simulink model "MPCtest1"  (Simulink 10.0)
settings: Solver=VariableStepDiscrete  StartTime=0.0  StopTime=30  FixedStep=0.01  RelTol=1e-3  EnableMultiTasking=on
libraries: Solver_SF x1, simulink x1
settings Model: Creator=xuwei  LastModifiedBy=Administrator
settings DataIOCC: LimitDataPoints=on  SignalLoggingSaveFormat=ModelDataLogs
settings OptimizationCC: ExpressionDepthLimit=2147483647
settings DebuggingCC: SolverPrmCheckMsg=warning  FcnCallInpInsideContextMsg=warning  StateNameClashWarn=warning
settings GRTTargetCC: GeneratePreprocessorConditionals=Disable all
settings ConfigComp: CovExternalEMLEnable=off
settings SimscapeCC: SimscapeNormalizeSystem=off
settings ConfigurationSet: Description=SimMechanics 2G

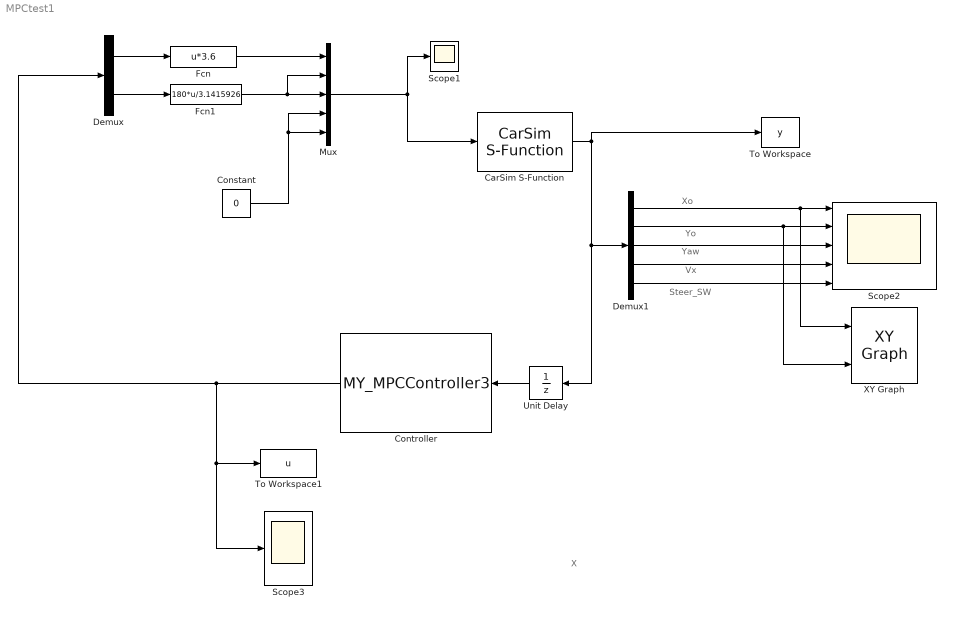
== system MPCtest1 ==
  note: Yo
  note: Xo
  note: Yaw
  note: Vx
  note: Steer_SW
  note: X
  CarSim S-Function : Solver_SF/CarSim S-Function  Priority=1  VehicleCode=i_i  SIMFILE=simfile
  Constant : Constant  Value=0
  Controller : S-Function  FunctionName=MY_MPCController3  SFunctionDeploymentMode=off  EnableBusSupport=off
  Demux : Demux  Outputs=2
  Demux1 : Demux  Outputs=5
  Fcn : Fcn  Expr=u*3.6
  Fcn1 : Fcn  Expr=180*u/3.1415926
  Mux : Mux  Inputs=5
  Scope1 : Scope
  Scope2 : Scope  NumInputPorts=5
  Scope3 : Scope
  To Workspace : ToWorkspace  VariableName=y  SaveFormat=Structure  SampleTime=-1
  To Workspace1 : ToWorkspace  VariableName=u  SaveFormat=Structure  SampleTime=-1
  Unit Delay : UnitDelay  SampleTime=-1  HasFrameUpgradeWarning=on
  XY Graph : simulink/Sinks/XY Graph  xmin=-100  xmax=200  ymin=-100  ymax=200  st=-1
  wires:
  Unit Delay/1 -> Controller/1
  Mux/1 -> CarSim S-Function/1, Scope1/1
  Constant/1 -> Mux/5, Mux/4
  Fcn/1 -> Mux/1
  Fcn1/1 -> Mux/2, Mux/3
  Demux/1 -> Fcn/1
  Demux/2 -> Fcn1/1
  Controller/1 -> Demux/1, Scope3/1, To Workspace1/1
  Demux1/1 -> XY Graph/1, Scope2/1
  Demux1/2 -> XY Graph/2, Scope2/2
  Demux1/3 -> Scope2/3
  Demux1/4 -> Scope2/4
  Demux1/5 -> Scope2/5
  CarSim S-Function/1 -> Unit Delay/1, Demux1/1, To Workspace/1
